simulink model "landing_control"  (R2014b)
settings: Solver=ode23t  StartTime=0.0  StopTime=3  MaxStep=1e-3  RelTol=1e-12  AbsTol=1e-9
values from neighbouring files (symbols this model uses):
  alpha0 = 90*pi/180    (= 1.57079632679)    [initialize_final.m]    (also in initialize_leafspring.m; initialize_linearspring.m)
  c = 2*eta*sqrt(m*k)    [initialize_final.m]    (also in initialize_leafspring.m = 170.5; initialize_linearspring.m = 2*eta*sqrt(m*k1); leafspring_test.m = 2*xi*sqrt(m*k))
  dx0 = 0    [initialize_final.m]    (also in initialize_leafspring.m; initialize_linearspring.m)
  dy0 = 0    [initialize_final.m]    (also in initialize_leafspring.m; initialize_linearspring.m)
  g = 9.81    [initialize_final.m]    (also in initialize_leafspring.m; initialize_linearspring.m; leafspring_test.m)
  k = m*(v1^2 + g*Lleg)/(lx^2)    [initialize_final.m]    (also in initialize_linearspring.m = 941; leafspring_test.m = (TE*2)/(x_des)^2)
  Lleg = 1    [initialize_final.m]    (also in initialize_leafspring.m = 0.7; initialize_linearspring.m)
  m = 8    [initialize_final.m]    (also in initialize_leafspring.m = 5; initialize_linearspring.m; leafspring_test.m = 5)
  x0 = []    [AnimSMR3.m]    (also in initialize_final.m = 2; initialize_leafspring.m = 2; initialize_linearspring.m = 2)
  y0 = (2*i)*Lleg    [initialize_final.m]    (also in initialize_leafspring.m = (2.5*i)*Lleg; initialize_linearspring.m)
libraries: simulink_extras x1
settings Model: Creator=hgeyer  LastModifiedBy=Avinash
settings SolverCC: AlgebraicLoopSolver=LineSearch
settings DataIOCC: SignalLoggingSaveFormat=ModelDataLogs
settings OptimizationCC: ExpressionDepthLimit=2147483647
settings DebuggingCC: UnderspecifiedInitializationDetection=Classic  MergeDetectMultiDrivingBlocksExec=none  MultiTaskDSMMsg=warning  MultiTaskCondExecSysMsg=none  FcnCallInpInsideContextMsg=EnableAllAsWarning  StateNameClashWarn=warning
settings RTWCC: IncludeERTFirstTime=on

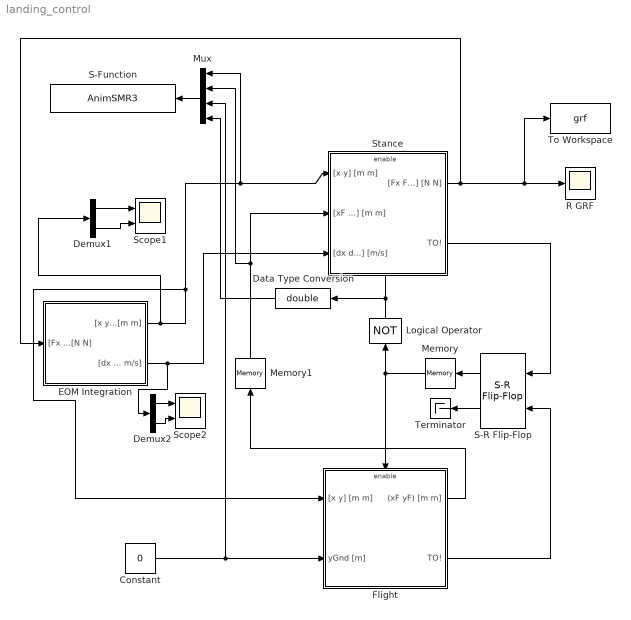
== system landing_control ==
  Constant : Constant  Value=0
  Data Type Conversion : DataTypeConversion  OutDataTypeStr=double
  Demux1 : Demux  Outputs=2
  Demux2 : Demux  Outputs=2
  EOM Integration : Subsystem
  Flight : Subsystem
  Logical Operator : Logic  Operator=NOT  AllPortsSameDT=off  OutDataTypeStr=boolean
  Memory : Memory  X0=1
  Memory1 : Memory  X0=[0 0]
  Mux : Mux
  R GRF : Scope
      settings: YMin=-1e+14  YMax=0
  S-Function : S-Function  FunctionName=AnimSMR3  Parameters=0.01  EnableBusSupport=off
  S-R Flip-Flop : simulink_extras/Flip Flops/S-R Flip-Flop  initial_condition=1
  Scope1 : Scope  NumInputPorts=2
      settings: YMin=3.8~-2.3e+254  YMax=4.2~0  SaveName=ScopeData8  MaxDataPoints=50000
  Scope2 : Scope  NumInputPorts=2
      settings: YMin=-1~-1.7e+206  YMax=1~1.7822e+190  SaveName=ScopeData5  MaxDataPoints=50000
  Stance : Subsystem
  Terminator : Terminator
  To Workspace : ToWorkspace  VariableName=grf  SaveFormat=Timeseries  SampleTime=-1
  wires:
  EOM Integration/1("[x y] [m m]") -> Demux1/1, Flight/1("[x y] [m m]"), Mux/1, Stance/1("[x y] [m m]")
  Stance/2(TO!) -> S-R Flip-Flop/1
  S-R Flip-Flop/1 -> Memory/1
  Logical Operator/1 -> Stance/Enable, Data Type Conversion/1
  Memory/1 -> Logical Operator/1, Flight/Enable
  Flight/2(TO!) -> S-R Flip-Flop/2
  Flight/1((xF yF) [m m]) -> Memory1/1
  Memory1/1 -> Mux/2, Stance/2("[xF yF] [m m]")
  Mux/1 -> S-Function/1
  S-R Flip-Flop/2 -> Terminator/1
  Stance/1("[Fx Fy] [N N]") -> To Workspace/1, R GRF/1, EOM Integration/1("[Fx Fy] [N N]")
  Constant/1 -> Flight/2(yGnd [m]), Mux/3
  Data Type Conversion/1 -> Mux/4
  Demux1/1 -> Scope1/1
  Demux1/2 -> Scope1/2
  EOM Integration/2("[dx dy] [m/s m/s]") -> Demux2/1, Stance/3("[dx dy] [m/s]")
  Demux2/1 -> Scope2/1
  Demux2/2 -> Scope2/2

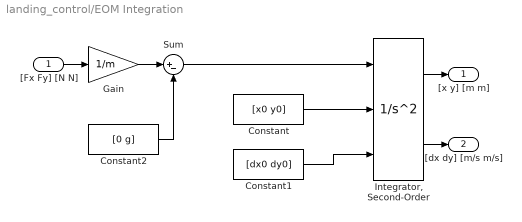
== system landing_control/EOM Integration ==
  "[Fx Fy] [N N]" : Inport
  Constant : Constant  Value=[x0 y0]
  Constant1 : Constant  Value=[dx0 dy0]
  Constant2 : Constant  Value=[0 g]
  Gain : Gain  Gain=1/m
  "Integrator, Second-Order" : SecondOrderIntegrator  ICSourceX=external  ICSourceDXDT=external
  Sum : Sum  Inputs=|+-
  "[x y] [m m]" : Outport
  "[dx dy] [m/s m/s]" : Outport  Port=2
  wires:
  Constant/1 -> "Integrator, Second-Order"/2
  Constant1/1 -> "Integrator, Second-Order"/3
  Gain/1 -> Sum/1
  Sum/1 -> "Integrator, Second-Order"/1
  Constant2/1 -> Sum/2
  "[Fx Fy] [N N]"/1 -> Gain/1
  "Integrator, Second-Order"/1 -> "[x y] [m m]"/1
  "Integrator, Second-Order"/2 -> "[dx dy] [m/s m/s]"/1

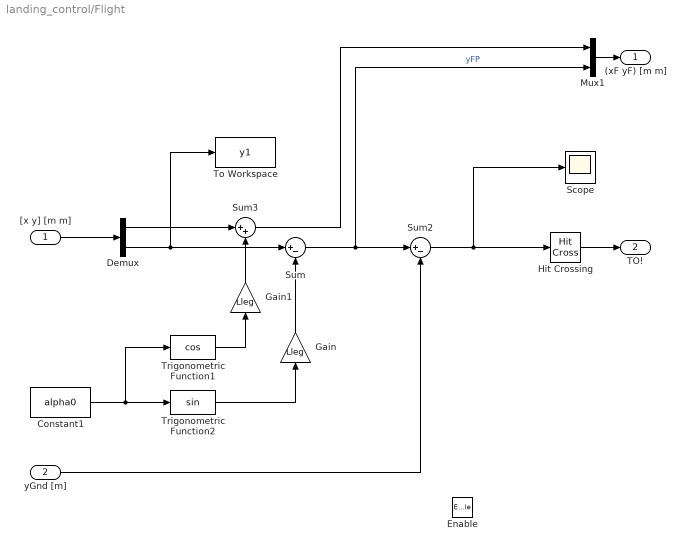
== system landing_control/Flight ==
  "[x y] [m m]" : Inport
  yGnd [m] : Inport  Port=2
  Enable : EnablePort  StatesWhenEnabling=reset
  Constant1 : Constant  Value=alpha0
  Demux : Demux  Outputs=2
  Gain : Gain  Gain=Lleg
  Gain1 : Gain  Gain=Lleg
  Hit Crossing : HitCross  HitCrossingDirection=falling
  Mux1 : Mux  Inputs=2
  Scope : Scope
      settings: SaveName=ScopeData6
  Sum : Sum  Inputs=|+-
  Sum2 : Sum  Inputs=|+-
  Sum3 : Sum  Inputs=|++
  To Workspace : ToWorkspace  VariableName=y1  SampleTime=-1
      settings: MaxDataPoints=1
  Trigonometric Function1 : Trigonometry  Operator=cos
  Trigonometric Function2 : Trigonometry
  (xF yF) [m m] : Outport  InitialOutput=0
  TO! : Outport  Port=2  OutputWhenDisabled=reset  InitialOutput=0
  wires:
  Hit Crossing/1 -> TO!/1
  Mux1/1 -> (xF yF) [m m]/1
  "[x y] [m m]"/1 -> Demux/1
  Demux/2 -> Sum/1, To Workspace/1
  Constant1/1 -> Trigonometric Function2/1, Trigonometric Function1/1
  Trigonometric Function2/1 -> Gain/1
  Gain/1 -> Sum/2
  Sum/1 -> Sum2/1, Mux1/2  "yFP"
  yGnd [m]/1 -> Sum2/2
  Sum2/1 -> Scope/1, Hit Crossing/1
  Trigonometric Function1/1 -> Gain1/1
  Gain1/1 -> Sum3/2
  Demux/1 -> Sum3/1
  Sum3/1 -> Mux1/1

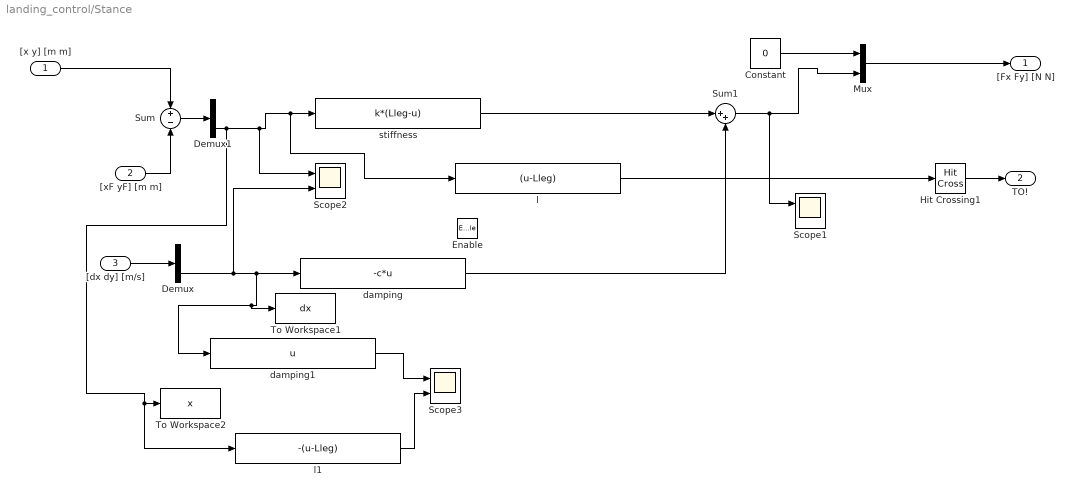
== system landing_control/Stance ==
  "[x y] [m m]" : Inport
  "[xF yF] [m m]" : Inport  Port=2
  "[dx dy] [m/s]" : Inport  Port=3
  Enable : EnablePort  StatesWhenEnabling=reset
  Constant : Constant  Value=0
  Demux : Demux  Outputs=2
  Demux1 : Demux  Outputs=2
  Hit Crossing1 : HitCross  HitCrossingDirection=rising
  Mux : Mux  Inputs=2
  Scope1 : Scope  NumInputPorts=2
      settings: YMin=-1.4e+23~-3.75e+24  YMax=-1.67772e+07~0  SaveName=ScopeData2  MaxDataPoints=50000
  Scope2 : Scope  NumInputPorts=2
      settings: YMin=-1.4e+23~-3.75e+24  YMax=-1.67772e+07~0  MaxDataPoints=50000
  Scope3 : Scope  NumInputPorts=2
      settings: YMin=-1.4e+23~-3.75e+24  YMax=-1.67772e+07~0  SaveName=ScopeData3  MaxDataPoints=50000
  Sum : Sum  Inputs=+-
  Sum1 : Sum  Inputs=|++
  To Workspace1 : ToWorkspace  VariableName=dx  SaveFormat=Timeseries  SampleTime=-1
  To Workspace2 : ToWorkspace  VariableName=x  SampleTime=-1
  damping : Fcn  Expr=-c*u
  damping1 : Fcn  Expr=u
  l : Fcn  Expr=(u-Lleg)
  l1 : Fcn  Expr=-(u-Lleg)
  stiffness : Fcn  Expr=k*(Lleg-u)
  "[Fx Fy] [N N]" : Outport  OutputWhenDisabled=reset  InitialOutput=[0 0]
  TO! : Outport  Port=2  OutputWhenDisabled=reset  InitialOutput=0
  wires:
  "[xF yF] [m m]"/1 -> Sum/2
  "[x y] [m m]"/1 -> Sum/1
  Hit Crossing1/1 -> TO!/1
  "[dx dy] [m/s]"/1 -> Demux/1
  Sum/1 -> Demux1/1
  Demux1/2 -> l1/1, To Workspace2/1, Scope2/1, l/1, stiffness/1
  stiffness/1 -> Sum1/1
  Demux/2 -> Scope2/2, To Workspace1/1, damping1/1, damping/1
  Sum1/1 -> Scope1/1, Mux/2
  Mux/1 -> "[Fx Fy] [N N]"/1
  Constant/1 -> Mux/1
  l/1 -> Hit Crossing1/1
  damping/1 -> Sum1/2
  damping1/1 -> Scope3/1
  l1/1 -> Scope3/2
